simulink model "InvPendStateFeedback_LQ"  (R2023b)
settings: Solver=VariableStepAuto  StartTime=0.0  StopTime=10  RelTol=1e-6
values from neighbouring files (symbols this model uses):
  A = [0      1              0           0 ... (first row only)    [InvPendModel.m]
  B = [     0 ... (first row only)    [InvPendModel.m]
  C = [1 0 0 0 ... (first row only)    [InvPendModel.m]
  D = [0 ... (first row only)    [InvPendModel.m]
  K = place(Ag,Bg,[-4 -3 -2.5 -2 -1])    [InvPendModel.m]
settings Model: Creator=alfredo  LastModifiedBy=roberto_ambrosino
settings SolverCC: AlgebraicLoopSolver=TrustRegion
settings DataIOCC: ReturnWorkspaceOutputs=off
settings DebuggingCC: UnconnectedInputMsg=warning  UnconnectedOutputMsg=warning  UnconnectedLineMsg=warning  ArithmeticOperatorsInVariantConditions=warning
settings ModelReferenceCC: EnableRefExpFcnMdlSchedulingChecks=on
settings SFSimCC: SimUseLocalCustomCode=off  CustomCodeUndefinedFunction=UseInterfaceOnly
settings RTWCC: RTWUseLocalCustomCode=off

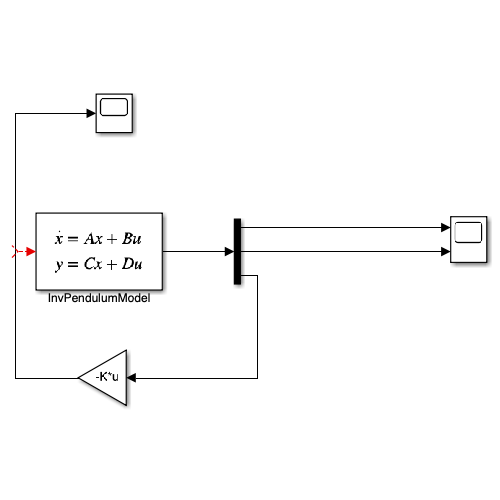
[thumbnail: Simulink's stored preview of the top-level diagram]
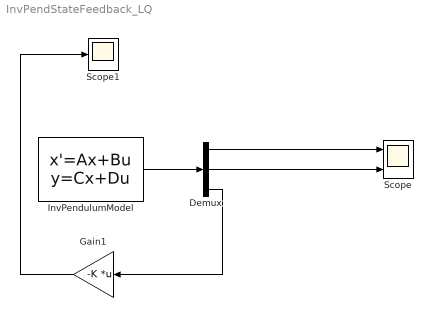
== system InvPendStateFeedback_LQ ==
  Demux : Demux  Outputs=[1 1 4]
  Gain1 : Gain  Gain=-K  Multiplication=Matrix(K*u)
  InvPendulumModel : StateSpace  A=A  B=B  C=[C;eye(4)]  D=[D;zeros(4,1)]  InitialCondition=[0.5 0 0.1 0]
  Scope : Scope  NumInputPorts=2
  Scope1 : Scope
  wires:
  Gain1/1 -> Scope1/1
  InvPendulumModel/1 -> Demux/1
  Demux/1 -> Scope/1
  Demux/2 -> Scope/2
  Demux/3 -> Gain1/1
  ? -> InvPendulumModel/1
